simulink model "HQEV_MiL_20160830_integrate_r2017a"  (Simulink 8.9)
settings: Solver=FixedStepDiscrete  StartTime=0.0  StopTime=inf  FixedStep=0.01  RelTol=1e-3  EnableMultiTasking=on
PostLoadFcn:
  | , if any(exist('dsrtsu_mdlpostloadfcn', 'file') == [2, 3, 6]), try dsrtsu_mdlpostloadfcn('Execute', bdroot); catch fprintf('Error in PostLoadFcn (dsrtsu_mdlpostloadfcn) for model "%s":\n %s\n', bdroot, lasterr); end, end,
values from neighbouring files (symbols this model uses):
  Bat_C_Ah = 36    [parameter_V1.mat]
  Bat_ocv_xIndex = [5 10 20 30 40 50 60 70 80 90 95]    [parameter_V1.mat]
  Bat_ocv_z = [329 332 340 345 347 351 358 372 377 386 391]    [parameter_V1.mat]
  Bat_R_ohm_z = [4.41 3.46 1.57 1.07 0.76 0.63 0.55 0.44 0.41 0.4 0.4 3.14 ... (66 elements, 11x6)]    [parameter_V1.mat]
  Bat_SOC_Init = 90    [parameter_V1.mat]
  Env_hum_pct_Ambient = 30    [parameter_V1.mat]
  Env_Slope_deg = 0    [parameter_V1.mat]
  Env_Temp_degC_Ambient = 25    [parameter_V1.mat]
  Env_v_kmph_HWind = 0    [parameter_V1.mat]
  Reducer_F_i = 7.23    [parameter_V1.mat]
  Reducer_R_i = 7.23    [parameter_V1.mat]
  Veh =     [parameter_V1.mat]
  Veh_A_m2_Fr = 2.246    [parameter_V1.mat]
  Veh_F_Brake =     [parameter_V1.mat]
  Veh_fac_AirDrag = 0.326    [parameter_V1.mat]
  Veh_fac_WhDragFrict_0 = 0.011    [parameter_V1.mat]
  Veh_g_mps2_C = 9.81    [parameter_V1.mat]
  Veh_GainBrake =     [parameter_V1.mat]
  Veh_h_m_COGHigh = 0.5    [parameter_V1.mat]
  Veh_J_kgm2_Wh = 1.3635    [parameter_V1.mat]
  Veh_L_m_AxlBas = 2.63    [parameter_V1.mat]
  Veh_M_kg = 1427    [parameter_V1.mat]
  Veh_mu_Brake = 0.4    [parameter_V1.mat]
  Veh_mu_Tyre =     [parameter_V1.mat]
  Veh_num_FrictPair = 8    [parameter_V1.mat]
  Veh_pct_Brk = 70    [parameter_V1.mat]
  Veh_r_dyn =     [parameter_V1.mat]
  Veh_r_m_BrkDisk = 0.136    [parameter_V1.mat]
  Veh_rho_kgpm3_Air = 1.2258    [parameter_V1.mat]
undefined symbols (not defined in the file or in its folder): DiscIntNeverNeededParam, p_bool_False_M, p_bool_True_M
libraries: BaseOperationLib_Browser x38, simulink x8, DTQC_lib x1, ERR_lib x1, MQM_lib x1, PTCL_lib x1, PUD_lib x1, TQD_lib x1, TQR_lib x1, VMM_lib x1, ACCA_lib x1, BBCA_lib x1
(part 12 of 15)

== system HQEV_MiL_20160830_integrate_r2017a/MiL/Test_Integration/Motor_FF/Motor/Motor/Uc_Management/RelayLogic ==
  note: 0:Open
      | 1:ShortCircle
      | 2:PreCharge
  note: DC Charge PreCharge
  note: AC Charge PreCharge
  Main_Pos : Inport
  PreCharg : Inport  Port=2
  Main_Neg : Inport  Port=3
  ChargePos : Inport  Port=4
  ChargeNeg : Inport  Port=5
  Charger_Status : Inport  Port=6
  Charger Working : Constant
  Combinatorial  Logic : CombinatorialLogic  TruthTable=[0;0;0;2;0;1;0;1]
  Logical Operator : Logic  AllPortsSameDT=off  OutDataTypeStr=boolean
  Logical Operator1 : Logic  Operator=OR  AllPortsSameDT=off  OutDataTypeStr=boolean
  Logical Operator2 : Logic  AllPortsSameDT=off  OutDataTypeStr=boolean
  Logical Operator3 : Logic  Operator=OR  AllPortsSameDT=off  OutDataTypeStr=boolean
  Logical Operator4 : Logic  Operator=NOT  AllPortsSameDT=off  OutDataTypeStr=boolean
  Mux : Mux  Inputs=3
  PreCharger : Constant  Value=2
  Relational Operator : RelationalOperator  Operator===  OutDataTypeStr=boolean  RndMeth=Nearest
  Switch : Switch  Criteria=u2 ~= 0
  Out1 : Outport
  wires:
  Mux/1 -> Combinatorial  Logic/1
  Main_Pos/1 -> Logical Operator1/1, Mux/1
  PreCharg/1 -> Logical Operator1/2, Mux/2
  Main_Neg/1 -> Mux/3
  ChargePos/1 -> Logical Operator/1
  ChargeNeg/1 -> Logical Operator/2
  Logical Operator1/1 -> Logical Operator2/1
  Logical Operator/1 -> Logical Operator2/2
  Charger_Status/1 -> Relational Operator/1
  Charger Working/1 -> Relational Operator/2
  Logical Operator2/1 -> Logical Operator3/1
  Relational Operator/1 -> Logical Operator3/2
  Switch/1 -> Out1/1
  Logical Operator3/1 -> Logical Operator4/1
  Logical Operator4/1 -> Switch/2
  PreCharger/1 -> Switch/3
  Combinatorial  Logic/1 -> Switch/1

== system HQEV_MiL_20160830_integrate_r2017a/MiL/Test_Integration/Motor_FF/Motor/Motor/Uc_Management/ShortCircle ==
  Bat_U : Inport
  Bus Creator : BusCreator  Inputs=2
  Constant : Constant  Value=1.0000e-006
  EM_C : Constant  Value=600
      settings: AttributesFormatString=Unit:muF
  F : Product  RndMeth=Zero
  RC : Product  RndMeth=Zero
  R_precharge : Constant  Value=20
      settings: AttributesFormatString=Unit:ohm
  Out1 : Outport
  wires:
  Bat_U/1 -> Bus Creator/1  "U_Term"
  EM_C/1 -> F/1
  Constant/1 -> F/2
  R_precharge/1 -> RC/1
  F/1 -> RC/2
  RC/1 -> Bus Creator/2  "RC"
  Bus Creator/1 -> Out1/1

== system HQEV_MiL_20160830_integrate_r2017a/MiL/Test_Integration/Motor_FF/Motor/Motor/eMotor/Electric Power ==
  n_Motor : Inport
  T_Motor : Inport  Port=2
  Bus Creator : BusCreator  Inputs=4
  Bus Selector : BusSelector  OutputSignals=n_Mot,T_Mot
  Motor Electric Power : Subsystem
  Motor Mechanical Power : Subsystem
  Motor System Efficiency : Lookup2D  RowIndex=[-2000,-1000,1000,2000]  ColumnIndex=[-200,-100,100,200]  Table=reshape([0.85,0.85,0.85,0.85,0.85,0.85,0.85,0.85,0.85,0.85,0.85,0.85,0.85,0.85,0.85,0.85],4,4)
  P_Motor_elec : Outport
  P_Motor_loss : Outport  Port=2
  wires:
  Motor Electric Power/1(EM1_pwr_elec) -> P_Motor_elec/1
  Bus Creator/1 -> Bus Selector/1, Motor Mechanical Power/1(In1), Motor Electric Power/1(In1)
  Bus Selector/1 -> Motor System Efficiency/1  "<n_Mot>"
  Bus Selector/2 -> Motor System Efficiency/2  "<T_Mot>"
  Motor Mechanical Power/1(EM_pwr_mech) -> Bus Creator/1  "P_Mech"
  Motor System Efficiency/1 -> Bus Creator/2  "eta"
  n_Motor/1 -> Bus Creator/3  "n_Mot"
  T_Motor/1 -> Bus Creator/4  "T_Mot"
  Motor Electric Power/2(EM1_pwr_loss) -> P_Motor_loss/1

== system HQEV_MiL_20160830_integrate_r2017a/MiL/Test_Integration/Motor_FF/Motor/Motor/eMotor/Motor Torque ==
  MCU1_trq_req : Inport
  Unit Delay : UnitDelay  SampleTime=-1
  T_Motor : Outport
  wires:
  MCU1_trq_req/1 -> Unit Delay/1
  Unit Delay/1 -> T_Motor/1

== system HQEV_MiL_20160830_integrate_r2017a/MiL/Test_Integration/Motor_RR/Motor/Motor1/Uc_Management/Open ==
  RapidDischargeEnable : Inport
  Uc : Inport  Port=2
  Bus Creator : BusCreator  Inputs=2
  Constant : Constant  Value=1.0000e-006
  Constant1 : Constant  Value=0
  EM_C : Constant  Value=600
      settings: AttributesFormatString=Unit:muF
  F : Product  RndMeth=Zero
  RC : Product  RndMeth=Zero
  R_precharge : Constant  Value=1000
      settings: AttributesFormatString=Unit:ohm
  Switch : Switch  Criteria=u2 ~= 0
  Out1 : Outport
  wires:
  EM_C/1 -> F/1
  Constant/1 -> F/2
  R_precharge/1 -> RC/1
  F/1 -> RC/2
  RC/1 -> Bus Creator/2  "RC"
  RapidDischargeEnable/1 -> Switch/2
  Uc/1 -> Switch/3
  Switch/1 -> Bus Creator/1  "U_Term"
  Constant1/1 -> Switch/1
  Bus Creator/1 -> Out1/1

== system HQEV_MiL_20160830_integrate_r2017a/MiL/Test_Integration/Motor_RR/Motor/Motor1/Uc_Management/PreCharg ==
  Bat_U : Inport
  Bus Creator : BusCreator  Inputs=2
  Constant : Constant  Value=1.0000e-006
  EM_C : Constant  Value=600
      settings: AttributesFormatString=Unit:muF
  F : Product  RndMeth=Zero
  RC : Product  RndMeth=Zero
  R_precharge : Constant  Value=55
      settings: AttributesFormatString=Unit:ohm
  Out : Outport
  wires:
  Bus Creator/1 -> Out/1
  Bat_U/1 -> Bus Creator/1  "U_Term"
  EM_C/1 -> F/1
  Constant/1 -> F/2
  R_precharge/1 -> RC/1
  F/1 -> RC/2
  RC/1 -> Bus Creator/2  "RC"

== system HQEV_MiL_20160830_integrate_r2017a/MiL/Test_Integration/Motor_RR/Motor/Motor1/Uc_Management/RelayLogic ==
  note: 0:Open
      | 1:ShortCircle
      | 2:PreCharge
  note: DC Charge PreCharge
  note: AC Charge PreCharge
  Main_Pos : Inport
  PreCharg : Inport  Port=2
  Main_Neg : Inport  Port=3
  ChargePos : Inport  Port=4
  ChargeNeg : Inport  Port=5
  Charger_Status : Inport  Port=6
  Charger Working : Constant
  Combinatorial  Logic : CombinatorialLogic  TruthTable=[0;0;0;2;0;1;0;1]
  Logical Operator : Logic  AllPortsSameDT=off  OutDataTypeStr=boolean
  Logical Operator1 : Logic  Operator=OR  AllPortsSameDT=off  OutDataTypeStr=boolean
  Logical Operator2 : Logic  AllPortsSameDT=off  OutDataTypeStr=boolean
  Logical Operator3 : Logic  Operator=OR  AllPortsSameDT=off  OutDataTypeStr=boolean
  Logical Operator4 : Logic  Operator=NOT  AllPortsSameDT=off  OutDataTypeStr=boolean
  Mux : Mux  Inputs=3
  PreCharger : Constant  Value=2
  Relational Operator : RelationalOperator  Operator===  OutDataTypeStr=boolean  RndMeth=Nearest
  Switch : Switch  Criteria=u2 ~= 0
  Out1 : Outport
  wires:
  Mux/1 -> Combinatorial  Logic/1
  Main_Pos/1 -> Logical Operator1/1, Mux/1
  PreCharg/1 -> Logical Operator1/2, Mux/2
  Main_Neg/1 -> Mux/3
  ChargePos/1 -> Logical Operator/1
  ChargeNeg/1 -> Logical Operator/2
  Logical Operator1/1 -> Logical Operator2/1
  Logical Operator/1 -> Logical Operator2/2
  Charger_Status/1 -> Relational Operator/1
  Charger Working/1 -> Relational Operator/2
  Logical Operator2/1 -> Logical Operator3/1
  Relational Operator/1 -> Logical Operator3/2
  Switch/1 -> Out1/1
  Logical Operator3/1 -> Logical Operator4/1
  Logical Operator4/1 -> Switch/2
  PreCharger/1 -> Switch/3
  Combinatorial  Logic/1 -> Switch/1

== system HQEV_MiL_20160830_integrate_r2017a/MiL/Test_Integration/Motor_RR/Motor/Motor1/Uc_Management/ShortCircle ==
  Bat_U : Inport
  Bus Creator : BusCreator  Inputs=2
  Constant : Constant  Value=1.0000e-006
  EM_C : Constant  Value=600
      settings: AttributesFormatString=Unit:muF
  F : Product  RndMeth=Zero
  RC : Product  RndMeth=Zero
  R_precharge : Constant  Value=20
      settings: AttributesFormatString=Unit:ohm
  Out1 : Outport
  wires:
  Bat_U/1 -> Bus Creator/1  "U_Term"
  EM_C/1 -> F/1
  Constant/1 -> F/2
  R_precharge/1 -> RC/1
  F/1 -> RC/2
  RC/1 -> Bus Creator/2  "RC"
  Bus Creator/1 -> Out1/1

== system HQEV_MiL_20160830_integrate_r2017a/MiL/Test_Integration/Motor_RR/Motor/Motor1/eMotor/Electric Power ==
  n_Motor : Inport
  T_Motor : Inport  Port=2
  Bus Creator : BusCreator  Inputs=4
  Bus Selector : BusSelector  OutputSignals=n_Mot,T_Mot
  Motor Electric Power : Subsystem
  Motor Mechanical Power : Subsystem
  Motor System Efficiency : Lookup2D  RowIndex=[-2000,-1000,1000,2000]  ColumnIndex=[-200,-100,100,200]  Table=reshape([0.85,0.85,0.85,0.85,0.85,0.85,0.85,0.85,0.85,0.85,0.85,0.85,0.85,0.85,0.85,0.85],4,4)
  P_Motor_elec : Outport
  P_Motor_loss : Outport  Port=2
  wires:
  Motor Electric Power/1(EM1_pwr_elec) -> P_Motor_elec/1
  Bus Creator/1 -> Bus Selector/1, Motor Mechanical Power/1(In1), Motor Electric Power/1(In1)
  Bus Selector/1 -> Motor System Efficiency/1  "<n_Mot>"
  Bus Selector/2 -> Motor System Efficiency/2  "<T_Mot>"
  Motor Mechanical Power/1(EM_pwr_mech) -> Bus Creator/1  "P_Mech"
  Motor System Efficiency/1 -> Bus Creator/2  "eta"
  n_Motor/1 -> Bus Creator/3  "n_Mot"
  T_Motor/1 -> Bus Creator/4  "T_Mot"
  Motor Electric Power/2(EM1_pwr_loss) -> P_Motor_loss/1

== system HQEV_MiL_20160830_integrate_r2017a/MiL/Test_Integration/Motor_RR/Motor/Motor1/eMotor/Motor Torque ==
  MCU1_trq_req : Inport
  Unit Delay : UnitDelay  SampleTime=-1
  T_Motor : Outport
  wires:
  MCU1_trq_req/1 -> Unit Delay/1
  Unit Delay/1 -> T_Motor/1

== system HQEV_MiL_20160830_integrate_r2017a/MiL/Test_Integration/Reducer_F/FinalDrive/FinalDrive/Subsystem/Backward ==
  T_in : Inport
  Divide : Product  Inputs=*/
  Efficiency : Subsystem
  Ground : Ground
  Ground1 : Ground
  Ground2 : Ground
  Product : Product  RndMeth=Zero
  ratio : Constant  Value=Reducer_F_i
  T_out : Outport
  wires:
  Ground/1 -> Efficiency/1(T_in)
  Ground1/1 -> Efficiency/2("Temp ")
  Ground2/1 -> Efficiency/3("Omega_in ")
  T_in/1 -> Divide/1
  Efficiency/1(eta) -> Divide/2
  Divide/1 -> Product/1
  Product/1 -> T_out/1
  ratio/1 -> Product/2

== system HQEV_MiL_20160830_integrate_r2017a/MiL/Test_Integration/Reducer_F/FinalDrive/FinalDrive/Subsystem/Derection ==
  n_Wheel : Inport
  T_in : Inport  Port=2
  Constant : Constant  Value=0
  Product : Product  RndMeth=Zero
  Relational Operator : RelationalOperator  OutDataTypeStr=boolean  RndMeth=Nearest
  derection : Outport
  wires:
  T_in/1 -> Product/2
  n_Wheel/1 -> Product/1
  Product/1 -> Relational Operator/1
  Constant/1 -> Relational Operator/2
  Relational Operator/1 -> derection/1

== system HQEV_MiL_20160830_integrate_r2017a/MiL/Test_Integration/Reducer_F/FinalDrive/FinalDrive/Subsystem/Forward ==
  T_in : Inport
  Efficiency : Subsystem
  Ground : Ground
  Ground1 : Ground
  Ground2 : Ground
  Product : Product  RndMeth=Zero
  Product1 : Product  RndMeth=Zero
  ratio : Constant  Value=Reducer_F_i
  T_out : Outport
  wires:
  Ground/1 -> Efficiency/1(T_in)
  Ground1/1 -> Efficiency/2("Temp ")
  Ground2/1 -> Efficiency/3("Omega_in ")
  T_in/1 -> Product/1
  Efficiency/1(eta) -> Product/2
  Product/1 -> Product1/1
  ratio/1 -> Product1/2
  Product1/1 -> T_out/1

== system HQEV_MiL_20160830_integrate_r2017a/MiL/Test_Integration/Reducer_R/FinalDrive/FinalDrive/Subsystem/Backward ==
  T_in : Inport
  Constant : Constant  Value=Reducer_R_i
  Divide : Product  Inputs=*/
  Efficiency : Subsystem
  Ground : Ground
  Ground1 : Ground
  Ground2 : Ground
  Product : Product  RndMeth=Zero
  T_out : Outport
  wires:
  Efficiency/1(eta) -> Divide/2
  T_in/1 -> Divide/1
  Ground2/1 -> Efficiency/3("Omega_in ")
  Ground1/1 -> Efficiency/2("Temp ")
  Ground/1 -> Efficiency/1(T_in)
  Divide/1 -> Product/1
  Constant/1 -> Product/2
  Product/1 -> T_out/1

== system HQEV_MiL_20160830_integrate_r2017a/MiL/Test_Integration/Reducer_R/FinalDrive/FinalDrive/Subsystem/Derection ==
  n_Wheel : Inport
  T_in : Inport  Port=2
  Constant : Constant  Value=0
  Product : Product  RndMeth=Zero
  Relational Operator : RelationalOperator  OutDataTypeStr=boolean  RndMeth=Nearest
  derection : Outport
  wires:
  Relational Operator/1 -> derection/1
  Constant/1 -> Relational Operator/2
  Product/1 -> Relational Operator/1
  n_Wheel/1 -> Product/1
  T_in/1 -> Product/2

== system HQEV_MiL_20160830_integrate_r2017a/MiL/Test_Integration/Reducer_R/FinalDrive/FinalDrive/Subsystem/Forward ==
  T_in : Inport
  Constant : Constant  Value=Reducer_R_i
  Efficiency : Subsystem
  Ground : Ground
  Ground1 : Ground
  Ground2 : Ground
  Product : Product  RndMeth=Zero
  Product1 : Product  RndMeth=Zero
  T_out : Outport
  wires:
  Efficiency/1(eta) -> Product/2
  T_in/1 -> Product/1
  Ground2/1 -> Efficiency/3("Omega_in ")
  Ground1/1 -> Efficiency/2("Temp ")
  Ground/1 -> Efficiency/1(T_in)
  Product/1 -> Product1/1
  Constant/1 -> Product1/2
  Product1/1 -> T_out/1

== system HQEV_MiL_20160830_integrate_r2017a/MiL/Test_Integration/Thermal/Thermal/Subsystem/Battery_Cooling_Circle/Battery ==
  note: CQ(T2-T1)=h[T0-(T2+T1)/2]
      | T2=(hT0+CQT1-T1h/2)/(CQ+h/2)
  note: h: forced convective heat transfer coefficient
  T_water_Inlet : Inport
  Q_water_Inlet : Inport  Port=2
  pwr_BatteryLoss : Inport  Port=3
  BatTempIndex : Inport  Port=4
  Bus Creator : BusCreator  Inputs=2
  Bus Creator1 : BusCreator  Inputs=2
  Bus Selector : BusSelector  OutputSignals=T
  Constant : Constant
  Forced Convective : Subsystem
  Free Convective : Subsystem
  Relational Operator : RelationalOperator  Operator=>  OutDataTypeStr=boolean  RndMeth=Nearest
  Switch : Switch  Criteria=u2 ~= 0
  Thermal_Mass : Subsystem
  T_Battery : Outport
  T_water_outlet : Outport  Port=2
  wires:
  Bus Selector/1 -> T_water_outlet/1  "<T>"
  Switch/1 -> Bus Selector/1
  Bus Creator1/1 -> Switch/3
  Free Convective/2(Q_water_outlet) -> Bus Creator1/2  "Q"
  Free Convective/1(T_water_outlet) -> Bus Creator1/1  "T"
  Bus Creator/1 -> Switch/1
  T_water_Inlet/1 -> Free Convective/2(T_water_inlet), Forced Convective/3(T_water_inlet)
  Q_water_Inlet/1 -> Forced Convective/2(Q_water_inlet), Free Convective/1(Q_water_inlet), Relational Operator/1
  Forced Convective/2(T_water_outlet) -> Bus Creator/1  "T"
  Forced Convective/3(Q_water_outlet) -> Bus Creator/2  "Q"
  Forced Convective/1(q_Water2Motor) -> Thermal_Mass/2(pwr_Water2Motor)
  pwr_BatteryLoss/1 -> Thermal_Mass/1(pwr_MotorLoss)
  Thermal_Mass/1(T_Motor) -> Forced Convective/1(T_Motor), T_Battery/1
  Constant/1 -> Relational Operator/2
  Relational Operator/1 -> Switch/2
  BatTempIndex/1 -> Thermal_Mass/3(BatTempIndex)

== system HQEV_MiL_20160830_integrate_r2017a/MiL/Test_Integration/Thermal/Thermal/Subsystem/Battery_Cooling_Circle/Chiller ==
  note: CQ(T2-T1)=h[T0-(T2+T1)/2]
      | T2=(hT0+CQT1-T1h/2)/(CQ+h/2)
  note: h: forced convective heat transfer coefficient
  Q_water_inlet : Inport
  T_water_inlet : Inport  Port=2
  AC_OnOff : Inport  Port=3
  Bus Creator : BusCreator  Inputs=2
  Bus Creator1 : BusCreator  Inputs=2
  Bus Selector : BusSelector  OutputSignals=T,Q
  Constant : Constant
  Forced Convective : Subsystem
  Free Convective : Subsystem
  Ground : Ground
  Relational Operator : RelationalOperator  Operator=>  OutDataTypeStr=boolean  RndMeth=Nearest
  Switch : Switch  Criteria=u2 ~= 0
  Q_water_outlet : Outport
  T_water_outlet : Outport  Port=2
  NULL : Outport  Port=3
  wires:
  Ground/1 -> NULL/1
  Bus Selector/2 -> Q_water_outlet/1  "<Q>"
  Bus Selector/1 -> T_water_outlet/1  "<T>"
  Switch/1 -> Bus Selector/1
  Bus Creator1/1 -> Switch/3
  Free Convective/2(Q_water_outlet) -> Bus Creator1/2  "Q"
  Free Convective/1(T_water_outlet) -> Bus Creator1/1  "T"
  Bus Creator/1 -> Switch/1
  Forced Convective/2(Q_water_outlet) -> Bus Creator/2  "Q"
  Forced Convective/1(T_water_outlet) -> Bus Creator/1  "T"
  T_water_inlet/1 -> Free Convective/2(T_water_inlet), Forced Convective/3(Temp_water_inlet)
  Q_water_inlet/1 -> Forced Convective/2(Q_water_inlet), Free Convective/1(Q_water_inlet), Relational Operator/1
  AC_OnOff/1 -> Forced Convective/1(AC_OnOff)
  Relational Operator/1 -> Switch/2
  Constant/1 -> Relational Operator/2

== system HQEV_MiL_20160830_integrate_r2017a/MiL/Test_Integration/Thermal/Thermal/Subsystem/Battery_Cooling_Circle/PTC ==
  note: CQ(T2-T1)=h[T0-(T2+T1)/2]
      | T2=(hT0+CQT1-T1h/2)/(CQ+h/2)
  note: h: forced convective heat transfer coefficient
  Q_water_inlet : Inport
  T_water_inlet : Inport  Port=2
  PWM_PTC_pct : Inport  Port=3
  Bus Creator : BusCreator  Inputs=2
  Bus Creator1 : BusCreator  Inputs=2
  Bus Selector : BusSelector  OutputSignals=T,Q
  Constant : Constant
  Forced Convective : Subsystem
  Free Convective : Subsystem
  Ground : Ground
  Relational Operator : RelationalOperator  Operator=>  OutDataTypeStr=boolean  RndMeth=Nearest
  Switch : Switch  Criteria=u2 ~= 0
  Q_water_outlet : Outport
  T_water_outlet : Outport  Port=2
  NULL : Outport  Port=3
  wires:
  Ground/1 -> NULL/1
  Bus Selector/2 -> Q_water_outlet/1  "<Q>"
  Bus Selector/1 -> T_water_outlet/1  "<T>"
  Switch/1 -> Bus Selector/1
  Bus Creator1/1 -> Switch/3
  Free Convective/2(Q_water_outlet) -> Bus Creator1/2  "Q"
  Free Convective/1(T_water_outlet) -> Bus Creator1/1  "T"
  Bus Creator/1 -> Switch/1
  Forced Convective/2(Q_water_outlet) -> Bus Creator/2  "Q"
  Forced Convective/1(T_water_outlet) -> Bus Creator/1  "T"
  T_water_inlet/1 -> Free Convective/2(T_water_inlet), Forced Convective/3(Temp_water_inlet)
  Q_water_inlet/1 -> Forced Convective/2(Q_water_inlet), Free Convective/1(Q_water_inlet), Relational Operator/1
  PWM_PTC_pct/1 -> Forced Convective/1(PWM_PTC_pct)
  Relational Operator/1 -> Switch/2
  Constant/1 -> Relational Operator/2

== system HQEV_MiL_20160830_integrate_r2017a/MiL/Test_Integration/Thermal/Thermal/Subsystem/Battery_Cooling_Circle/Pump_Battery ==
  PWM_Battery : Inport
  T_Water_Inlet : Inport  Port=2
  Divide : Product  Inputs=*/
  L/min : Constant  Value=30
  L/s : Constant  Value=60
  Product1 : Product  RndMeth=Zero
  Product2 : Product  RndMeth=Zero
  Product3 : Product  RndMeth=Zero
  kg/s : Constant
  pct-1 : Constant  Value=0.01
  Q_Water_outlet : Outport
  T_Water_outlet : Outport  Port=2
  wires:
  T_Water_Inlet/1 -> T_Water_outlet/1
  L/min/1 -> Product1/2
  PWM_Battery/1 -> Product2/1
  pct-1/1 -> Product2/2
  Product2/1 -> Product1/1
  Product1/1 -> Divide/1
  L/s/1 -> Divide/2
  Divide/1 -> Product3/1
  kg/s/1 -> Product3/2
  Product3/1 -> Q_Water_outlet/1

== system HQEV_MiL_20160830_integrate_r2017a/MiL/Test_Integration/Thermal/Thermal/Subsystem/Motor_Cooling_Circle/Charger ==
  note: h: forced convective heat transfer coefficient
  note: CQ(T2-T1)=h[T0-(T2+T1)/2]
      | T2=(hT0+CQT1-T1h/2)/(CQ+h/2)
  Q_water_Inlet : Inport
  T_water_Inlet : Inport  Port=2
  pwr_ChargerLoss : Inport  Port=3
  Bus Creator : BusCreator  Inputs=2
  Bus Creator1 : BusCreator  Inputs=2
  Bus Selector : BusSelector  OutputSignals=T,Q
  Constant : Constant
  Forced Convective : Subsystem
  Free Convective : Subsystem
  Relational Operator : RelationalOperator  Operator=>  OutDataTypeStr=boolean  RndMeth=Nearest
  Switch : Switch  Criteria=u2 ~= 0
  Thermal_Mass : Subsystem
  T_Charger : Outport
  Q_water_outlet : Outport  Port=2
  T_water_outlet : Outport  Port=3
  wires:
  Bus Selector/2 -> Q_water_outlet/1  "<Q>"
  Bus Selector/1 -> T_water_outlet/1  "<T>"
  Switch/1 -> Bus Selector/1
  Bus Creator1/1 -> Switch/3
  Free Convective/2(Q_water_outlet) -> Bus Creator1/2  "Q"
  Free Convective/1(T_water_outlet) -> Bus Creator1/1  "T"
  Bus Creator/1 -> Switch/1
  T_water_Inlet/1 -> Free Convective/2(T_water_inlet), Forced Convective/3(T_water_inlet)
  Q_water_Inlet/1 -> Forced Convective/2(Q_water_inlet), Free Convective/1(Q_water_inlet), Relational Operator/1
  Forced Convective/2(T_water_outlet) -> Bus Creator/1  "T"
  Forced Convective/3(Q_water_outlet) -> Bus Creator/2  "Q"
  Forced Convective/1(q_Water2Motor) -> Thermal_Mass/2(pwr_Water2Motor)
  pwr_ChargerLoss/1 -> Thermal_Mass/1(pwr_MotorLoss)
  Thermal_Mass/1(T_Motor) -> Forced Convective/1(T_Motor), T_Charger/1
  Constant/1 -> Relational Operator/2
  Relational Operator/1 -> Switch/2

== system HQEV_MiL_20160830_integrate_r2017a/MiL/Test_Integration/Thermal/Thermal/Subsystem/Motor_Cooling_Circle/DCDC ==
  note: h: forced convective heat transfer coefficient
  note: CQ(T2-T1)=h[T0-(T2+T1)/2]
      | T2=(hT0+CQT1-T1h/2)/(CQ+h/2)
  T_water_Inlet : Inport
  Q_water_Inlet : Inport  Port=2
  pwr_DCDCLoss : Inport  Port=3
  Bus Creator : BusCreator  Inputs=2
  Bus Creator1 : BusCreator  Inputs=2
  Bus Selector : BusSelector  OutputSignals=T
  Constant : Constant
  Forced Convective : Subsystem
  Free Convective : Subsystem
  Relational Operator : RelationalOperator  Operator=>  OutDataTypeStr=boolean  RndMeth=Nearest
  Switch : Switch  Criteria=u2 ~= 0
  Thermal_Mass : Subsystem
  T_DCDC : Outport
  T_water_outlet : Outport  Port=2
  wires:
  Bus Selector/1 -> T_water_outlet/1  "<T>"
  Switch/1 -> Bus Selector/1
  Bus Creator1/1 -> Switch/3
  Free Convective/2(Q_water_outlet) -> Bus Creator1/2  "Q"
  Free Convective/1(T_water_outlet) -> Bus Creator1/1  "T"
  Bus Creator/1 -> Switch/1
  T_water_Inlet/1 -> Free Convective/2(T_water_inlet), Forced Convective/3(T_water_inlet)
  Q_water_Inlet/1 -> Forced Convective/2(Q_water_inlet), Free Convective/1(Q_water_inlet), Relational Operator/1
  Forced Convective/2(T_water_outlet) -> Bus Creator/1  "T"
  Forced Convective/3(Q_water_outlet) -> Bus Creator/2  "Q"
  Forced Convective/1(q_Water2Motor) -> Thermal_Mass/2(pwr_Water2Motor)
  pwr_DCDCLoss/1 -> Thermal_Mass/1(pwr_MotorLoss)
  Thermal_Mass/1(T_Motor) -> Forced Convective/1(T_Motor), T_DCDC/1
  Constant/1 -> Relational Operator/2
  Relational Operator/1 -> Switch/2

== system HQEV_MiL_20160830_integrate_r2017a/MiL/Test_Integration/Thermal/Thermal/Subsystem/Motor_Cooling_Circle/Motor_F ==
  note: CQ(T2-T1)=h[T0-(T2+T1)/2]
      | T2=(hT0+CQT1-T1h/2)/(CQ+h/2)
  note: h: forced convective heat transfer coefficient
  T_water_Inlet : Inport
  Q_water_Inlet : Inport  Port=2
  pwr_MotorLoss : Inport  Port=3
  Bus Creator : BusCreator  Inputs=2
  Bus Creator1 : BusCreator  Inputs=2
  Bus Selector : BusSelector  OutputSignals=T,Q
  Constant : Constant
  Forced Convective : Subsystem
  Free Convective : Subsystem
  Relational Operator : RelationalOperator  Operator=>  OutDataTypeStr=boolean  RndMeth=Nearest
  Switch : Switch  Criteria=u2 ~= 0
  Thermal_Mass : Subsystem
  T_Motor : Outport
  Q_water_outlet : Outport  Port=2
  T_water_outlet : Outport  Port=3
  wires:
  Bus Selector/2 -> Q_water_outlet/1  "<Q>"
  Bus Selector/1 -> T_water_outlet/1  "<T>"
  Switch/1 -> Bus Selector/1
  Bus Creator1/1 -> Switch/3
  Free Convective/2(Q_water_outlet) -> Bus Creator1/2  "Q"
  Free Convective/1(T_water_outlet) -> Bus Creator1/1  "T"
  Bus Creator/1 -> Switch/1
  T_water_Inlet/1 -> Free Convective/2(T_water_inlet), Forced Convective/3(T_water_inlet)
  Q_water_Inlet/1 -> Forced Convective/2(Q_water_inlet), Free Convective/1(Q_water_inlet), Relational Operator/1
  Forced Convective/2(T_water_outlet) -> Bus Creator/1  "T"
  Forced Convective/3(Q_water_outlet) -> Bus Creator/2  "Q"
  Forced Convective/1(q_Water2Motor) -> Thermal_Mass/2(pwr_Water2Motor)
  pwr_MotorLoss/1 -> Thermal_Mass/1(pwr_MotorLoss)
  Thermal_Mass/1(T_Motor) -> Forced Convective/1(T_Motor), T_Motor/1
  Constant/1 -> Relational Operator/2
  Relational Operator/1 -> Switch/2

== system HQEV_MiL_20160830_integrate_r2017a/MiL/Test_Integration/Thermal/Thermal/Subsystem/Motor_Cooling_Circle/Motor_R ==
  note: h: forced convective heat transfer coefficient
  note: CQ(T2-T1)=h[T0-(T2+T1)/2]
      | T2=(hT0+CQT1-T1h/2)/(CQ+h/2)
  T_water_Inlet : Inport
  Q_water_Inlet : Inport  Port=2
  pwr_MotorLoss : Inport  Port=3
  Bus Creator : BusCreator  Inputs=2
  Bus Creator1 : BusCreator  Inputs=2
  Bus Selector : BusSelector  OutputSignals=T,Q
  Constant : Constant
  Forced Convective : Subsystem
  Free Convective : Subsystem
  Relational Operator : RelationalOperator  Operator=>  OutDataTypeStr=boolean  RndMeth=Nearest
  Switch : Switch  Criteria=u2 ~= 0
  Thermal_Mass : Subsystem
  Q_water_outlet : Outport
  T_water_outlet : Outport  Port=2
  T_Motor : Outport  Port=3
  wires:
  Bus Selector/2 -> Q_water_outlet/1  "<Q>"
  Bus Selector/1 -> T_water_outlet/1  "<T>"
  Switch/1 -> Bus Selector/1
  Bus Creator1/1 -> Switch/3
  Free Convective/2(Q_water_outlet) -> Bus Creator1/2  "Q"
  Free Convective/1(T_water_outlet) -> Bus Creator1/1  "T"
  Bus Creator/1 -> Switch/1
  T_water_Inlet/1 -> Free Convective/2(T_water_inlet), Forced Convective/3(T_water_inlet)
  Q_water_Inlet/1 -> Forced Convective/2(Q_water_inlet), Free Convective/1(Q_water_inlet), Relational Operator/1
  Forced Convective/2(T_water_outlet) -> Bus Creator/1  "T"
  Forced Convective/3(Q_water_outlet) -> Bus Creator/2  "Q"
  Forced Convective/1(q_Water2Motor) -> Thermal_Mass/2(pwr_Water2Motor)
  pwr_MotorLoss/1 -> Thermal_Mass/1(pwr_MotorLoss)
  Thermal_Mass/1(T_Motor) -> Forced Convective/1(T_Motor), T_Motor/1
  Constant/1 -> Relational Operator/2
  Relational Operator/1 -> Switch/2

== system HQEV_MiL_20160830_integrate_r2017a/MiL/Test_Integration/Thermal/Thermal/Subsystem/Motor_Cooling_Circle/Multiple_Input_Joint ==
  Q1 : Inport
  T1 : Inport  Port=2
  Q2 : Inport  Port=3
  T2 : Inport  Port=4
  Add : Sum
  Add1 : Sum
  Divide : Product  Inputs=*/
  Product : Product  RndMeth=Zero
  Product1 : Product  RndMeth=Zero
  Saturation : Saturate  UpperLimit=inf  LowerLimit=0.1
  Q0 : Outport
  T0 : Outport  Port=2
  wires:
  Q1/1 -> Product/1, Add1/1
  T1/1 -> Product/2
  Q2/1 -> Product1/1, Add1/2
  T2/1 -> Product1/2
  Product/1 -> Add/1
  Product1/1 -> Add/2
  Add/1 -> Divide/1
  Add1/1 -> Saturation/1
  Divide/1 -> T0/1
  Saturation/1 -> Divide/2, Q0/1

== system HQEV_MiL_20160830_integrate_r2017a/MiL/Test_Integration/Thermal/Thermal/Subsystem/Motor_Cooling_Circle/Pump_F ==
  T_Water_Inlet : Inport
  PWM_Pump1 : Inport  Port=2
  Divide : Product  Inputs=*/
  L/min : Constant  Value=30
  L/s : Constant  Value=60
  Product : Product  RndMeth=Zero
  Product1 : Product  RndMeth=Zero
  Product2 : Product  RndMeth=Zero
  kg/s : Constant
  pct-1 : Constant  Value=0.01
  T_Water_outlet : Outport
  Q_Water_outlet : Outport  Port=2
  wires:
  T_Water_Inlet/1 -> T_Water_outlet/1
  L/min/1 -> Product/2
  PWM_Pump1/1 -> Product1/1
  pct-1/1 -> Product1/2
  Product1/1 -> Product/1
  Product/1 -> Divide/1
  L/s/1 -> Divide/2
  Divide/1 -> Product2/1
  kg/s/1 -> Product2/2
  Product2/1 -> Q_Water_outlet/1

== system HQEV_MiL_20160830_integrate_r2017a/MiL/Test_Integration/Thermal/Thermal/Subsystem/Motor_Cooling_Circle/Pump_R ==
  T_Water_Inlet : Inport
  PWM_Pump2 : Inport  Port=2
  Divide : Product  Inputs=*/
  L/min : Constant  Value=30
  L/s : Constant  Value=60
  Product : Product  RndMeth=Zero
  Product1 : Product  RndMeth=Zero
  Product2 : Product  RndMeth=Zero
  kg/s : Constant
  pct-1 : Constant  Value=0.01
  T_Water_outlet : Outport
  Q_Water_outlet : Outport  Port=2
  wires:
  T_Water_Inlet/1 -> T_Water_outlet/1
  L/min/1 -> Product/2
  PWM_Pump2/1 -> Product1/1
  pct-1/1 -> Product1/2
  Product1/1 -> Product/1
  Product/1 -> Divide/1
  L/s/1 -> Divide/2
  Divide/1 -> Product2/1
  kg/s/1 -> Product2/2
  Product2/1 -> Q_Water_outlet/1

== system HQEV_MiL_20160830_integrate_r2017a/MiL/Test_Integration/Thermal/Thermal/Subsystem/Motor_Cooling_Circle/Radiator ==
  note: h: forced convective heat transfer coefficient
  note: CQ(T2-T1)=h[T0-(T2+T1)/2]
      | T2=(hT0+CQT1-T1h/2)/(CQ+h/2)
  Q_water_inlet : Inport
  T_water_inlet : Inport  Port=2
  PWM_Fan : Inport  Port=3
  Bus Creator : BusCreator  Inputs=2
  Bus Creator1 : BusCreator  Inputs=2
  Bus Selector : BusSelector  OutputSignals=T,Q
  Constant1 : Constant
  Forced Convective : Subsystem
  Free Convective : Subsystem
  Ground : Ground
  Relational Operator : RelationalOperator  Operator=>  OutDataTypeStr=boolean  RndMeth=Nearest
  Switch : Switch  Criteria=u2 ~= 0
  Q_water_outlet : Outport
  T_water_outlet : Outport  Port=2
  NULL : Outport  Port=3
  wires:
  Q_water_inlet/1 -> Free Convective/1(Q_water_inlet), Forced Convective/3(T_water_inlet), Forced Convective/2(Q_water_inlet), Relational Operator/1
  T_water_inlet/1 -> Free Convective/2(T_water_inlet)
  Bus Creator/1 -> Switch/1
  Free Convective/1(T_water_outlet) -> Bus Creator1/1  "T"
  Free Convective/2(Q_water_outlet) -> Bus Creator1/2  "Q"
  Bus Creator1/1 -> Switch/3
  Switch/1 -> Bus Selector/1
  Bus Selector/1 -> T_water_outlet/1  "<T>"
  Bus Selector/2 -> Q_water_outlet/1  "<Q>"
  Ground/1 -> NULL/1
  PWM_Fan/1 -> Forced Convective/1(PWM_Fan)
  Forced Convective/1(T_water_outlet) -> Bus Creator/1  "T"
  Forced Convective/2(Q_water_outlet) -> Bus Creator/2  "Q"
  Constant1/1 -> Relational Operator/2
  Relational Operator/1 -> Switch/2

== system HQEV_MiL_20160830_integrate_r2017a/MiL/Test_Integration/Vehicle/Vehicle/Vehicle/Resistance Torque/Sigmoid-Function ==
  x1 : Inport
  Ctrl : Inport  Port=2
  x2 : Inport  Port=3
  Constant1 : Constant  Value=Offset
  Constant2 : Constant
  Constant3 : Constant
  Damping : Gain  Gain=Damping  SaturateOnIntegerOverflow=on  OutDataTypeStr=Inherit: Same as input  ParamDataTypeStr=Inherit: Same as input
  Damping1 : Gain  Gain=-Damping  SaturateOnIntegerOverflow=on  OutDataTypeStr=Inherit: Same as input  ParamDataTypeStr=Inherit: Same as input
  Math Function : Math  Operator=reciprocal  SaturateOnIntegerOverflow=on
  Math Function1 : Math  SaturateOnIntegerOverflow=on
  Math Function2 : Math  Operator=reciprocal  SaturateOnIntegerOverflow=on
  Math Function3 : Math  SaturateOnIntegerOverflow=on
  Product : Product  SaturateOnIntegerOverflow=on  OutDataTypeStr=Inherit: Same as first input
  Product1 : Product  SaturateOnIntegerOverflow=on  OutDataTypeStr=Inherit: Same as first input
  Sum : Sum  Inputs=|+-  SaturateOnIntegerOverflow=on
  Sum1 : Sum  Inputs=++|  SaturateOnIntegerOverflow=on
  Sum2 : Sum  Inputs=++|  SaturateOnIntegerOverflow=on
  Sum3 : Sum  SaturateOnIntegerOverflow=on
  y : Outport
  wires:
  Sum3/1 -> y/1
  Math Function2/1 -> Product1/2
  Math Function/1 -> Product/2
  Product1/1 -> Sum3/2
  Product/1 -> Sum3/1
  x2/1 -> Product1/1
  x1/1 -> Product/1
  Damping1/1 -> Math Function3/1
  Sum2/1 -> Math Function2/1
  Constant3/1 -> Sum2/1
  Math Function3/1 -> Sum2/2
  Sum1/1 -> Math Function/1
  Constant2/1 -> Sum1/1
  Math Function1/1 -> Sum1/2
  Damping/1 -> Math Function1/1
  Sum/1 -> Damping1/1, Damping/1
  Constant1/1 -> Sum/2
  Ctrl/1 -> Sum/1

== system HQEV_MiL_20160830_integrate_r2017a/MiL/Test_Integration/Vehicle/Vehicle/Vehicle/Resistance Torque/air_drag ==
  v_Veh [km/h] : Inport
  v_Hwind [m/s] : Inport  Port=2
  Gain : Gain  Gain=0.5  SaturateOnIntegerOverflow=on  OutDataTypeStr=Inherit: Same as input  ParamDataTypeStr=Inherit: Same as input
  Gain1 : Gain  Gain=1/3.6  SaturateOnIntegerOverflow=on  OutDataTypeStr=Inherit: Same as input  ParamDataTypeStr=Inherit: Same as input
  Math Function : Math  Operator=square  SaturateOnIntegerOverflow=on
  Product : Product  Inputs=4  SaturateOnIntegerOverflow=on  InputSameDT=on  OutDataTypeStr=Inherit: Same as first input
  Sum1 : Sum  SaturateOnIntegerOverflow=on  InputSameDT=on  OutDataTypeStr=Inherit: Same as first input
  air density : Constant  Value=Veh_rho_kgpm3_Air
  air drag coefficient : Constant  Value=Veh_fac_AirDrag
  front aerea cross section : Constant  Value=Veh_A_m2_Fr
  F_AirDrag [N] : Outport
  wires:
  Gain1/1 -> Sum1/1
  air density/1 -> Gain/1
  v_Veh [km/h]/1 -> Gain1/1
  v_Hwind [m/s]/1 -> Sum1/2
  Sum1/1 -> Math Function/1
  Math Function/1 -> Product/4
  Product/1 -> F_AirDrag [N]/1
  front aerea cross section/1 -> Product/1
  Gain/1 -> Product/3
  air drag coefficient/1 -> Product/2

== system HQEV_MiL_20160830_integrate_r2017a/MiL/Test_Integration/Vehicle/Vehicle/Vehicle/Resistance Torque/slope_drag ==
  m [kg] : Inport
  phi_Slope [deg] : Inport  Port=2
  " " : Gain  Gain=-1  SaturateOnIntegerOverflow=on  OutDataTypeStr=Inherit: Same as input  ParamDataTypeStr=Inherit: Same as input
  Product4 : Product  SaturateOnIntegerOverflow=on  InputSameDT=on  OutDataTypeStr=Inherit: Same as first input
  Trigonometric Function : Trigonometry
  grad to radiant : Gain  Gain=pi/180  SaturateOnIntegerOverflow=on  OutDataTypeStr=Inherit: Same as input  ParamDataTypeStr=Inherit: Same as input
  gravity constant : Gain  Gain=Veh_g_mps2_C  SaturateOnIntegerOverflow=on  OutDataTypeStr=Inherit: Same as input  ParamDataTypeStr=Inherit: Same as input
  F_Slope [N] : Outport
  wires:
  " "/1 -> F_Slope [N]/1
  m [kg]/1 -> gravity constant/1
  gravity constant/1 -> Product4/1
  Trigonometric Function/1 -> Product4/2
  phi_Slope [deg]/1 -> grad to radiant/1
  grad to radiant/1 -> Trigonometric Function/1
  Product4/1 -> " "/1

== system HQEV_MiL_20160830_integrate_r2017a/MiL/Test_Integration/Vehicle/Vehicle/Vehicle/Resistance Torque/wheel_drag ==
  phi_Slope [deg] : Inport
  m [kg] : Inport  Port=2
  v_Veh [m/s] : Inport  Port=3
  Abs : Abs  SaturateOnIntegerOverflow=on
  Constant : Constant  Value=Veh_fac_WhDragFrict_0
  Product4 : Product  Inputs=3  SaturateOnIntegerOverflow=on  InputSameDT=on  OutDataTypeStr=Inherit: Same as first input
  Terminator : Terminator
  Trigonometric Function : Trigonometry  Operator=cos
  grad to radiant : Gain  Gain=2*pi/360  SaturateOnIntegerOverflow=on  OutDataTypeStr=Inherit: Same as input  ParamDataTypeStr=Inherit: Same as input
  gravity constant : Gain  Gain=Veh_g_mps2_C  SaturateOnIntegerOverflow=on  OutDataTypeStr=Inherit: Same as input  ParamDataTypeStr=Inherit: Same as input
  " F_Wh_drag [N]" : Outport
  wires:
  v_Veh [m/s]/1 -> Abs/1
  Product4/1 -> " F_Wh_drag [N]"/1
  m [kg]/1 -> gravity constant/1
  gravity constant/1 -> Product4/2
  Trigonometric Function/1 -> Product4/3
  phi_Slope [deg]/1 -> grad to radiant/1
  grad to radiant/1 -> Trigonometric Function/1
  Constant/1 -> Product4/1
  Abs/1 -> Terminator/1

== system HQEV_MiL_20160830_integrate_r2017a/MiL/Test_Integration/Vehicle/Vehicle/Vehicle/Wheel Torque/Brake ==
  Sig_Brake [%] : Inport
  Omega_wh [rad/s] : Inport  Port=2
  " 1" : Gain  Gain=-1  OutDataTypeStr=Inherit: Same as input  ParamDataTypeStr=Inherit: Same as input
  Constant : Constant  Value=20
  Constant13 : Constant  Value=Veh_mu_Brake
  Constant7 : Constant  Value=Veh_r_m_BrkDisk
  Constant8 : Constant  Value=Veh_num_FrictPair
  Divide : Product  Inputs=*/
  Product1 : Product  SaturateOnIntegerOverflow=on  InputSameDT=on  OutDataTypeStr=Inherit: Same as first input
  Product7 : Product  SaturateOnIntegerOverflow=on  InputSameDT=on  OutDataTypeStr=Inherit: Same as first input
  Trigonometric Function : Trigonometry  Operator=tanh
  brake characteristic : Lookup  InputValues=Veh_F_Brake.x1  Table=Veh_F_Brake.z  LookUpMeth=Interpolation-Use End Values  SaturateOnIntegerOverflow=on
  brake servo : Gain  Gain=Veh_GainBrake.z  SaturateOnIntegerOverflow=on  OutDataTypeStr=Inherit: Same as input  ParamDataTypeStr=Inherit: Same as input
  direction : Product  SaturateOnIntegerOverflow=on  InputSameDT=on  OutDataTypeStr=Inherit: Same as first input
  direction2 : Product  SaturateOnIntegerOverflow=on  InputSameDT=on  OutDataTypeStr=Inherit: Same as first input
  T_Brake [Nm] : Outport
  wires:
  Divide/1 -> Trigonometric Function/1
  Constant8/1 -> direction2/1
  Product7/1 -> direction2/2  "friction torque"
  Product1/1 -> Product7/2  "friction force"
  brake servo/1 -> Product1/2
  Constant13/1 -> Product1/1
  brake characteristic/1 -> brake servo/1  "normal force"
  Constant7/1 -> Product7/1
  direction2/1 -> direction/1
  " 1"/1 -> direction/2
  Sig_Brake [%]/1 -> brake characteristic/1
  direction/1 -> T_Brake [Nm]/1
  Omega_wh [rad/s]/1 -> Divide/1
  Trigonometric Function/1 -> " 1"/1
  Constant/1 -> Divide/2

== system HQEV_MiL_20160830_integrate_r2017a/MiL/Test_Integration/Vehicle/Vehicle/Vehicle/Wheel Torque/Wheel_Torque ==
  T_maxFront [Nm] : Inport
  T_maxRear [Nm] : Inport  Port=2
  T_inFront [Nm] : Inport  Port=3
  T_inRear [Nm] : Inport  Description=Input torque [Nm]  Port=4
  T_Brake [Nm] : Inport  Port=5
  Abs : Abs
  Abs1 : Abs
  Brake_ProportionalFront : Gain  Gain=Veh_pct_Brk/100
  Brake_ProportionalRear : Gain  Gain=(100-Veh_pct_Brk)/100
  MinMax : MinMax  Inputs=2
  MinMax1 : MinMax  Inputs=2
  Product : Product  RndMeth=Zero
  Product1 : Product  RndMeth=Zero
  Sign : Signum
  Sign1 : Signum
  Sum1 : Sum
  Sum2 : Sum
  Sum3 : Sum
  T_Wheel_lim [Nm] : Outport
  wires:
  MinMax/1 -> Product/1
  T_maxFront [Nm]/1 -> MinMax/2
  Sign/1 -> Product/2
  Sum2/1 -> Sign/1, Abs/1
  Abs/1 -> MinMax/1
  MinMax1/1 -> Product1/1
  T_maxRear [Nm]/1 -> MinMax1/2
  Sign1/1 -> Product1/2
  Sum3/1 -> Abs1/1, Sign1/1
  Abs1/1 -> MinMax1/1
  T_Brake [Nm]/1 -> Brake_ProportionalFront/1, Brake_ProportionalRear/1
  Brake_ProportionalFront/1 -> Sum2/2
  Product1/1 -> Sum1/2
  Sum1/1 -> T_Wheel_lim [Nm]/1
  Product/1 -> Sum1/1
  Brake_ProportionalRear/1 -> Sum3/1
  T_inFront [Nm]/1 -> Sum2/1
  T_inRear [Nm]/1 -> Sum3/2

== system HQEV_MiL_20160830_integrate_r2017a/MiL/Test_Integration/Vehicle/Vehicle/Vehicle/Wheel Torque/maximal_wheel_torque ==
  phi_Slope [deg] : Inport
  acc_Vehicle [m/s^2] : Inport  Port=2
  m [kg] : Inport  Port=3
  F_to_T : Subsystem
  F_to_T_ : Subsystem
  Normal_force : Subsystem
  T_maxFront [Nm] : Outport
  T_maxRear [Nm] : Outport  Port=2
  wires:
  F_to_T_/1(T_max [Nm]) -> T_maxFront [Nm]/1
  Normal_force/2(F_normalRear [N]) -> F_to_T/1(F_normal [N])
  m [kg]/1 -> Normal_force/3(m [kg])
  Normal_force/1(F_normalFront [N]) -> F_to_T_/1(F_normal [N])
  phi_Slope [deg]/1 -> Normal_force/2(phi_Slope [deg])
  acc_Vehicle [m/s^2]/1 -> Normal_force/1(acc_Vehicle [m/s^2])
  F_to_T/1(T_max [Nm]) -> T_maxRear [Nm]/1

== system HQEV_MiL_20160830_integrate_r2017a/MiL/Test_Integration/BMS/BMS/BMS/BMS/Charge_Control/AC Charge connect ==
  SOC : Inport
  Bat_temp : Inport  Port=2
  HCU_ChargePermission : Inport  Port=3
  HCU_ChargeHeatingPermission : Inport  Port=4
  Constant{1..5,7..8,10,12} (9 alike) : Constant  Value=0
  Constant11 : Constant  Value=400
  Constant13 : Constant
  Constant6 : Constant  Value=400
  Constant9 : Constant  Value=95
  Data Type Conversion : DataTypeConversion  OutDataTypeStr=double
  Logical Operator : Logic  AllPortsSameDT=off  OutDataTypeStr=boolean
  Relational Operator : RelationalOperator  Operator=<  OutDataTypeStr=boolean  RndMeth=Nearest
  Relational Operator1 : RelationalOperator  Operator=>  OutDataTypeStr=boolean  RndMeth=Nearest
  Switch{1..4} (4 alike) : Switch  Criteria=u2 ~= 0
  BMS ChargeRequest : Outport
  BMS_ChargeStationOutputCurrent : Outport  Port=2
  BMS_ChargeStationOutputVoltage : Outport  Port=3
  BMS_InstantPowerConsumption : Outport  Port=4
  BMS_ChargeStationParameterConfigStatus : Outport  Port=5
  BMS_ChargeStationStatus : Outport  Port=6
  BMS_RemainingChargeTime : Outport  Port=7
  BMS_InsulationMonitorWarning : Outport  Port=8
  BMS_ChargeStationHandShakeStatus : Outport  Port=9
  BMS_ChargeStatus : Outport  Port=10
  wires:
  SOC/1 -> Relational Operator/1
  Constant9/1 -> Relational Operator/2
  Bat_temp/1 -> Relational Operator1/1
  Constant10/1 -> Relational Operator1/2
  Relational Operator/1 -> Logical Operator/1
  Relational Operator1/1 -> Logical Operator/2
  Constant1/1 -> BMS_ChargeStationOutputCurrent/1
  Switch3/1 -> BMS_ChargeStationOutputVoltage/1
  Constant3/1 -> BMS_InstantPowerConsumption/1
  Constant4/1 -> BMS_ChargeStationParameterConfigStatus/1
  Constant5/1 -> BMS_ChargeStationStatus/1
  Constant6/1 -> BMS_RemainingChargeTime/1
  Constant7/1 -> BMS_InsulationMonitorWarning/1
  Constant8/1 -> BMS_ChargeStationHandShakeStatus/1
  Logical Operator/1 -> Data Type Conversion/1
  Data Type Conversion/1 -> BMS ChargeRequest/1
  Switch2/1 -> BMS_ChargeStatus/1
  HCU_ChargePermission/1 -> Switch2/2, Switch4/2
  Constant13/1 -> Switch2/1, Switch1/1
  Switch1/1 -> Switch2/3
  HCU_ChargeHeatingPermission/1 -> Switch1/2, Switch3/2
  Constant12/1 -> Switch1/3
  Constant11/1 -> Switch3/1, Switch4/1
  Constant2/1 -> Switch4/3
  Switch4/1 -> Switch3/3

== system HQEV_MiL_20160830_integrate_r2017a/MiL/Test_Integration/BMS/BMS/BMS/BMS/Charge_Control/Connection_Check ==
  CC : Inport
  CC2 : Inport  Port=2
  Add : Sum
  Constant : Constant  Value=0
  Constant1 : Constant  Value=2
  Constant2 : Constant
  Constant3 : Constant  Value=0
  Constant4 : Constant  Value=0
  Logical Operator : Logic  AllPortsSameDT=off  OutDataTypeStr=boolean
  Switch : Switch  Criteria=u2 ~= 0
  Switch1 : Switch  Criteria=u2 ~= 0
  Switch2 : Switch  Criteria=u2 ~= 0  OutDataTypeStr=uint8
  Out1 : Outport
  wires:
  CC/1 -> Switch/2, Logical Operator/2
  Constant/1 -> Switch/3
  Constant1/1 -> Switch/1
  CC2/1 -> Switch1/2, Logical Operator/1
  Constant2/1 -> Switch1/1
  Constant3/1 -> Switch1/3
  Switch/1 -> Add/1
  Switch1/1 -> Add/2
  Add/1 -> Switch2/3
  Logical Operator/1 -> Switch2/2
  Constant4/1 -> Switch2/1
  Switch2/1 -> Out1/1

== system HQEV_MiL_20160830_integrate_r2017a/MiL/Test_Integration/BMS/BMS/BMS/BMS/Charge_Control/DC Charge connect ==
  CC2 : Inport
  SOC : Inport  Port=2
  Bat_temp : Inport  Port=3
  HCU_ChargePermission : Inport  Port=4
  HCU_ChargeHeatingPermission : Inport  Port=5
  Constant : Constant  Value=95
  Constant{1,4,6..8,12} (6 alike) : Constant  Value=0
  Constant11 : Constant  Value=10
  Constant13 : Constant
  Constant3 : Constant  Value=2
  Constant5 : Constant  Value=360
  Constant9 : Constant  Value=2
  Data Type Conversion : DataTypeConversion  OutDataTypeStr=double
  Logical Operator : Logic  AllPortsSameDT=off  OutDataTypeStr=boolean
  Relational Operator : RelationalOperator  Operator=<  OutDataTypeStr=boolean  RndMeth=Nearest
  Relational Operator1 : RelationalOperator  Operator=>  OutDataTypeStr=boolean  RndMeth=Nearest
  Switch{,1..5} (6 alike) : Switch  Criteria=u2 ~= 0
  kW : Constant  Value=0.5
  min : Constant  Value=400
  work : Constant
  BMS ChargeRequest : Outport
  BMS_ChargeStationOutputCurrent : Outport  Port=2
  BMS_ChargeStationOutputVoltage : Outport  Port=3
  BMS_InstantPowerConsumption : Outport  Port=4
  BMS_ChargeStationParameterConfigStatus : Outport  Port=5
  BMS_ChargeStationStatus : Outport  Port=6
  BMS_RemainingChargeTime : Outport  Port=7
  BMS_InsulationMonitorWarning : Outport  Port=8
  BMS_ChargeStationHandShakeStatus : Outport  Port=9
  BMS_ChargeStatus : Outport  Port=10
  wires:
  SOC/1 -> Relational Operator/1
  Constant/1 -> Relational Operator/2
  Bat_temp/1 -> Relational Operator1/1
  Constant1/1 -> Relational Operator1/2
  Relational Operator/1 -> Logical Operator/1
  Relational Operator1/1 -> Logical Operator/2
  Logical Operator/1 -> Data Type Conversion/1
  kW/1 -> BMS_InstantPowerConsumption/1
  work/1 -> BMS_ChargeStationStatus/1
  min/1 -> BMS_RemainingChargeTime/1
  Constant4/1 -> BMS_InsulationMonitorWarning/1
  Switch1/1 -> BMS_ChargeStationHandShakeStatus/1
  Constant3/1 -> Switch/1
  Constant7/1 -> Switch/3
  Switch/1 -> BMS_ChargeStationParameterConfigStatus/1
  Constant8/1 -> Switch1/3
  Constant9/1 -> Switch1/1
  Data Type Conversion/1 -> BMS ChargeRequest/1
  Constant11/1 -> BMS_ChargeStationOutputCurrent/1
  Switch3/1 -> BMS_ChargeStatus/1, Switch/2
  HCU_ChargePermission/1 -> Switch3/2, Switch5/2
  Constant13/1 -> Switch3/1, Switch2/1
  Switch2/1 -> Switch3/3
  HCU_ChargeHeatingPermission/1 -> Switch2/2, Switch4/2
  Constant12/1 -> Switch2/3
  CC2/1 -> Switch1/2
  Constant5/1 -> Switch4/1, Switch5/1
  Switch4/1 -> BMS_ChargeStationOutputVoltage/1
  Switch5/1 -> Switch4/3
  Constant6/1 -> Switch5/3

== system HQEV_MiL_20160830_integrate_r2017a/MiL/Test_Integration/BMS/BMS/BMS/BMS/Charge_Control/Disconnect ==
  Constant{,1..9} (10 alike) : Constant  Value=0
  BMS ChargeRequest : Outport
  BMS_ChargeStationOutputCurrent : Outport  Port=2
  BMS_ChargeStationOutputVoltage : Outport  Port=3
  BMS_InstantPowerConsumption : Outport  Port=4
  BMS_ChargeStationParameterConfigStatus : Outport  Port=5
  BMS_ChargeStationStatus : Outport  Port=6
  BMS_RemainingChargeTime : Outport  Port=7
  BMS_InsulationMonitorWarning : Outport  Port=8
  BMS_ChargeStationHandShakeStatus : Outport  Port=9
  BMS_ChargeStatus : Outport  Port=10
  wires:
  Constant/1 -> BMS ChargeRequest/1
  Constant1/1 -> BMS_ChargeStationOutputCurrent/1
  Constant2/1 -> BMS_ChargeStationOutputVoltage/1
  Constant3/1 -> BMS_InstantPowerConsumption/1
  Constant4/1 -> BMS_ChargeStationParameterConfigStatus/1
  Constant5/1 -> BMS_ChargeStationStatus/1
  Constant6/1 -> BMS_RemainingChargeTime/1
  Constant7/1 -> BMS_InsulationMonitorWarning/1
  Constant8/1 -> BMS_ChargeStationHandShakeStatus/1
  Constant9/1 -> BMS_ChargeStatus/1

== system HQEV_MiL_20160830_integrate_r2017a/MiL/Test_Integration/BMS/BMS/BMS/BMS/Relay_Control/Relay ==
  In1 : Inport
  Add : Sum
  Data Type Conversion : DataTypeConversion  OutDataTypeStr=boolean
  Data Type Conversion1 : DataTypeConversion  OutDataTypeStr=double
  Product : Product  RndMeth=Zero
  Rounding Function : Rounding  Operator=round
  Subtract : Sum  Inputs=+-
  Unit Delay2 : UnitDelay  SampleTime=-1
  tao : Constant
  Out1 : Outport
  wires:
  Subtract/1 -> Product/2
  In1/1 -> Data Type Conversion1/1
  tao/1 -> Product/1
  Product/1 -> Add/1
  Unit Delay2/1 -> Rounding Function/1, Subtract/2, Add/2
  Data Type Conversion/1 -> Out1/1
  Add/1 -> Unit Delay2/1
  Rounding Function/1 -> Data Type Conversion/1
  Data Type Conversion1/1 -> Subtract/1

== system HQEV_MiL_20160830_integrate_r2017a/MiL/Test_Integration/BMS/BMS/BMS/BMS/Relay_Control/Relay1 ==
  In1 : Inport
  Add : Sum
  Data Type Conversion : DataTypeConversion  OutDataTypeStr=boolean
  Data Type Conversion1 : DataTypeConversion  OutDataTypeStr=double
  Product : Product  RndMeth=Zero
  Rounding Function : Rounding  Operator=round
  Subtract : Sum  Inputs=+-
  Unit Delay2 : UnitDelay  SampleTime=-1
  tao : Constant
  Out1 : Outport
  wires:
  Rounding Function/1 -> Data Type Conversion/1
  Add/1 -> Unit Delay2/1
  Data Type Conversion/1 -> Out1/1
  Unit Delay2/1 -> Add/2, Subtract/2, Rounding Function/1
  Product/1 -> Add/1
  tao/1 -> Product/1
  In1/1 -> Data Type Conversion1/1
  Subtract/1 -> Product/2
  Data Type Conversion1/1 -> Subtract/1

== system HQEV_MiL_20160830_integrate_r2017a/MiL/Test_Integration/BMS/BMS/BMS/BMS/Relay_Control/Relay2 ==
  In1 : Inport
  Add : Sum
  Data Type Conversion : DataTypeConversion  OutDataTypeStr=boolean
  Data Type Conversion1 : DataTypeConversion  OutDataTypeStr=double
  Product : Product  RndMeth=Zero
  Rounding Function : Rounding  Operator=round
  Subtract : Sum  Inputs=+-
  Unit Delay2 : UnitDelay  SampleTime=-1
  tao : Constant
  Out1 : Outport
  wires:
  Subtract/1 -> Product/2
  In1/1 -> Data Type Conversion1/1
  tao/1 -> Product/1
  Product/1 -> Add/1
  Unit Delay2/1 -> Rounding Function/1, Subtract/2, Add/2
  Data Type Conversion/1 -> Out1/1
  Add/1 -> Unit Delay2/1
  Rounding Function/1 -> Data Type Conversion/1
  Data Type Conversion1/1 -> Subtract/1

== system HQEV_MiL_20160830_integrate_r2017a/MiL/Test_Integration/BMS/BMS/BMS/BMS/Relay_Control/Relay3 ==
  In1 : Inport
  Add : Sum
  Data Type Conversion : DataTypeConversion  OutDataTypeStr=boolean
  Data Type Conversion1 : DataTypeConversion  OutDataTypeStr=double
  Product : Product  RndMeth=Zero
  Rounding Function : Rounding  Operator=round
  Subtract : Sum  Inputs=+-
  Unit Delay2 : UnitDelay  SampleTime=-1
  tao : Constant
  Out1 : Outport
  wires:
  Rounding Function/1 -> Data Type Conversion/1
  Add/1 -> Unit Delay2/1
  Data Type Conversion/1 -> Out1/1
  Unit Delay2/1 -> Add/2, Subtract/2, Rounding Function/1
  Product/1 -> Add/1
  tao/1 -> Product/1
  In1/1 -> Data Type Conversion1/1
  Subtract/1 -> Product/2
  Data Type Conversion1/1 -> Subtract/1
